simulink model "wrm"  (R2015a)
settings: Solver=ode45  StartTime=0.0  StopTime=10.0  RelTol=1e-3
settings Model: Creator=rojas-j  LastModifiedBy=rojas-j

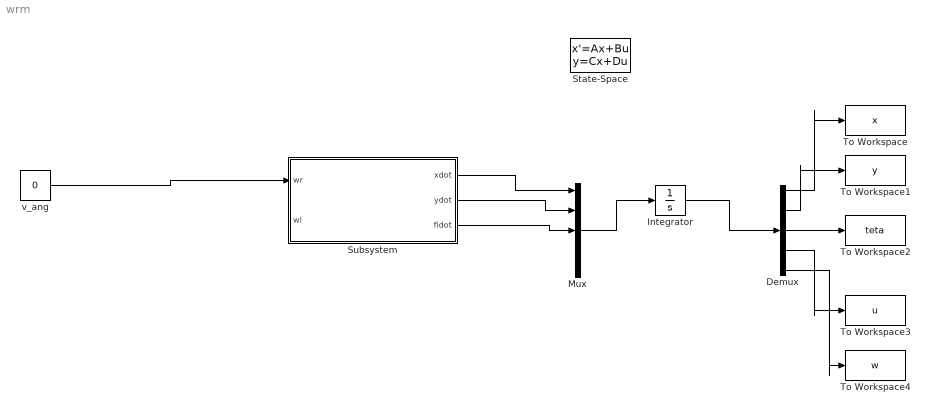
== system wrm ==
  Demux : Demux  Outputs=5
  Integrator : Integrator
  Mux : Mux  Inputs=5
  State-Space : StateSpace  X0=0
  Subsystem : Subsystem
  To Workspace : ToWorkspace  VariableName=x  SaveFormat=Timeseries  SampleTime=-1
  To Workspace1 : ToWorkspace  VariableName=y  SaveFormat=Timeseries  SampleTime=-1
  To Workspace2 : ToWorkspace  VariableName=teta  SaveFormat=Timeseries  SampleTime=-1
  To Workspace3 : ToWorkspace  VariableName=u  SaveFormat=Timeseries  SampleTime=-1
  To Workspace4 : ToWorkspace  VariableName=w  SaveFormat=Timeseries  SampleTime=-1
  v_ang : Constant  Value=0
  wires:
  v_ang/1 -> Subsystem/1(wr)
  Subsystem/1(xdot) -> Mux/1
  Subsystem/2(ydot) -> Mux/2
  Subsystem/3(fidot) -> Mux/3
  ? -> Mux/4
  ? -> Mux/5
  Mux/1 -> Integrator/1
  Integrator/1 -> Demux/1
  Demux/1 -> To Workspace/1
  Demux/2 -> To Workspace1/1
  Demux/3 -> To Workspace2/1
  Demux/4 -> To Workspace3/1
  Demux/5 -> To Workspace4/1

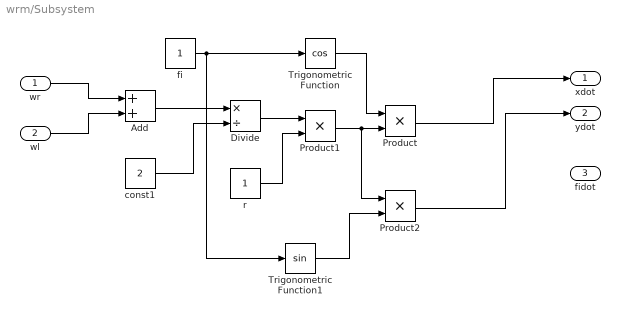
== system wrm/Subsystem ==
  wr : Inport
  wl : Inport  Port=2
  Add : Sum
  Divide : Product  Inputs=*/
  Product : Product
  Product1 : Product
  Product2 : Product
  Trigonometric Function : Trigonometry  Operator=cos
  Trigonometric Function1 : Trigonometry
  const1 : Constant  Value=2
  fi : Constant
  r : Constant
  xdot : Outport
  ydot : Outport  Port=2
  fidot : Outport  Port=3
  wires:
  wr/1 -> Add/1
  wl/1 -> Add/2
  Add/1 -> Divide/1
  const1/1 -> Divide/2
  Divide/1 -> Product1/1
  r/1 -> Product1/2
  fi/1 -> Trigonometric Function1/1, Trigonometric Function/1
  Trigonometric Function/1 -> Product/1
  Product1/1 -> Product2/1, Product/2
  Product/1 -> xdot/1
  Trigonometric Function1/1 -> Product2/2
  Product2/1 -> ydot/1
